simulink model "soc_pmsm_dualcpu_foc"  (R2023b)
settings: Solver=VariableStepAuto  StartTime=0.0  StopTime=.6  RelTol=1e-3  EnableMultiTasking=on
InitFcn:
  | soc_mcb_pmsm_foc_sensorless_f28379d_data;
model workspace (MAT data in the model file):
  mwTaskManagerKernelLatency = 0
values from neighbouring files (symbols this model uses):
  inverter = mcb_SetInverterParameters('BoostXL-DRV8305')    [soc_mcb_pmsm_foc_sensorless_f28379d_data.m]
  pmsm = mcb_SetPMSMMotorParameters('custom')    [soc_mcb_pmsm_foc_sensorless_f28379d_data.m]
  PU_System = mcb_SetPUSystem(pmsm,inverter)    [soc_mcb_pmsm_foc_sensorless_f28379d_data.m]
  PWM_frequency = 20e3    (= 20000)    [soc_mcb_pmsm_foc_sensorless_f28379d_data.m]
  Ts_motor = T_pwm/2    (= 2.5e-05)    [soc_mcb_pmsm_foc_sensorless_f28379d_data.m]
undefined symbols (not defined in the file or in its folder): D1, D2, Down, m, n, P, Up
libraries: fl_lib x50, nesl_utility x15, ee_lib x11, peripheralslib x5, procinterlib x2, proctasklib x2, mcbplantlib x1, mcbpositiondecoderlib x1, autolibpmsmexterior x1
(part 2 of 2)

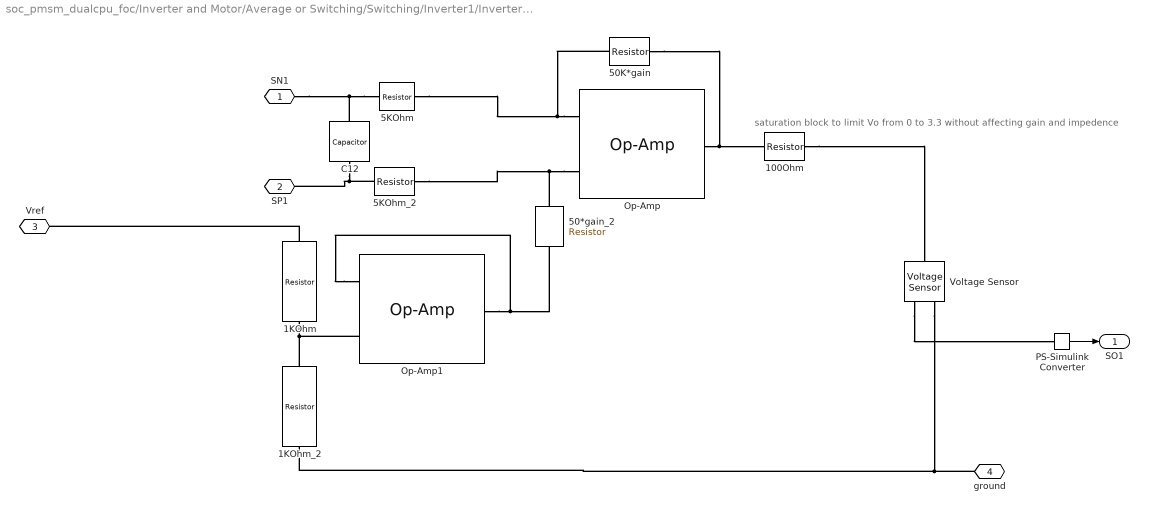
== system soc_pmsm_dualcpu_foc/Inverter and Motor/Average or Switching/Switching/Inverter1/Inverter/Current sense2 ==
  note: saturation block to limit Vo from 0 to 3.3 without affecting gain and impedence
  100Ohm : fl_lib/Electrical/Electrical Elements/Resistor  R=100 Ohm  i_specify=off  i_priority=None  i=0 A  i_nominal_specify=off  i_nominal_unit=A  i_nominal_value=1  v_specify=off  v_priority=None  v=0 V  v_nominal_specify=off  v_nominal_unit=V  v_nominal_value=1
  1KOhm : fl_lib/Electrical/Electrical Elements/Resistor  R=1 kOhm  i_specify=off  i_priority=None  i=0 A  i_nominal_specify=off  i_nominal_unit=A  i_nominal_value=1  v_specify=off  v_priority=None  v=0 V  v_nominal_specify=off  v_nominal_unit=V  v_nominal_value=1
  1KOhm_2 : fl_lib/Electrical/Electrical Elements/Resistor  R=1 kOhm  i_specify=off  i_priority=None  i=0 A  i_nominal_specify=off  i_nominal_unit=A  i_nominal_value=1  v_specify=off  v_priority=None  v=0 V  v_nominal_specify=off  v_nominal_unit=V  v_nominal_value=1
  50*gain_2 : fl_lib/Electrical/Electrical Elements/Resistor  R=50*inverter.ADCGain kOhm  i_specify=off  i_priority=None  i=0 A  i_nominal_specify=off  i_nominal_unit=A  i_nominal_value=1  v_specify=off  v_priority=None  v=0 V  v_nominal_specify=off  v_nominal_unit=V  v_nominal_value=1
  50K*gain : fl_lib/Electrical/Electrical Elements/Resistor  R=50*inverter.ADCGain kOhm  i_specify=off  i_priority=None  i=0 A  i_nominal_specify=off  i_nominal_unit=A  i_nominal_value=1  v_specify=off  v_priority=None  v=0 V  v_nominal_specify=off  v_nominal_unit=V  v_nominal_value=1
  5KOhm : fl_lib/Electrical/Electrical Elements/Resistor  R=5 kOhm  i_specify=off  i_priority=None  i=0 A  i_nominal_specify=off  i_nominal_unit=A  i_nominal_value=1  v_specify=off  v_priority=None  v=0 V  v_nominal_specify=off  v_nominal_unit=V  v_nominal_value=1
  5KOhm_2 : fl_lib/Electrical/Electrical Elements/Resistor  R=5 kOhm  i_specify=off  i_priority=None  i=0 A  i_nominal_specify=off  i_nominal_unit=A  i_nominal_value=1  v_specify=off  v_priority=None  v=0 V  v_nominal_specify=off  v_nominal_unit=V  v_nominal_value=1
  C12 : fl_lib/Electrical/Electrical Elements/Capacitor  c=1000 pF  r=1e-6 Ohm  g=0 1/Ohm  i_specify=off  i_priority=None  i=0 A  i_nominal_specify=off  i_nominal_unit=A  i_nominal_value=1  v_specify=off  v_priority=None  v=0 V  v_nominal_specify=off  v_nominal_unit=V  v_nominal_value=1  vc_specify=off  vc_priority=High  vc=0 V  vc_nominal_specify=off  vc_nominal_unit=V  vc_nominal_value=1
  Op-Amp : fl_lib/Electrical/Electrical Elements/Op-Amp  outI_specify=off  outI_priority=None  outI=0 A  outI_nominal_specify=off  outI_nominal_unit=A  outI_nominal_value=1
  Op-Amp1 : fl_lib/Electrical/Electrical Elements/Op-Amp  outI_specify=off  outI_priority=None  outI=0 A  outI_nominal_specify=off  outI_nominal_unit=A  outI_nominal_value=1
  PS-Simulink Converter : nesl_utility/PS-Simulink Converter  PhysicalDomain=network_engine_domain  SubClassName=ps_output  LeftPortType=input  RightPortType=output  PseudoPeriodic=off  Frequencies=[]  VectorFormat=1-D array  Unit=V  AffineConversion=off
  Voltage Sensor : fl_lib/Electrical/Electrical Sensors/Voltage Sensor
  SN1 : PMIOPort  Side=Left
  SP1 : PMIOPort  Port=2  Side=Left
  Vref : PMIOPort  Port=3  Side=Left
  ground : PMIOPort  Port=4  Side=Right
  SO1 : Outport  VectorParamsAs1DForOutWhenUnconnected=off
  wires:
  PS-Simulink Converter/1 -> SO1/1
  connections:
  100Ohm/RConn1 -- Voltage Sensor/LConn1
  Voltage Sensor/RConn1 -- PS-Simulink Converter/LConn1
  Voltage Sensor/RConn2 -- ground/RConn1 -- 1KOhm_2/RConn1
  5KOhm/LConn1 -- C12/LConn1 -- SN1/RConn1
  SP1/RConn1 -- C12/RConn1 -- 5KOhm_2/LConn1
  1KOhm/LConn1 -- Vref/RConn1
  Op-Amp/LConn1 -- 50*gain_2/LConn1 -- 5KOhm_2/RConn1
  Op-Amp1/LConn2 -- 50*gain_2/RConn1 -- Op-Amp1/RConn1
  Op-Amp/LConn2 -- 50K*gain/LConn1 -- 5KOhm/RConn1
  50K*gain/RConn1 -- 100Ohm/LConn1 -- Op-Amp/RConn1
  1KOhm/RConn1 -- Op-Amp1/LConn1 -- 1KOhm_2/LConn1
